simulink model "FlexibleJoint_PD"  (R2019b)
settings: Solver=VariableStepAuto  StartTime=0.0  StopTime=10  RelTol=1e-3
libraries: simulink x3, robotcorelib x1
settings Model: Creator=USER  LastModifiedBy=USER

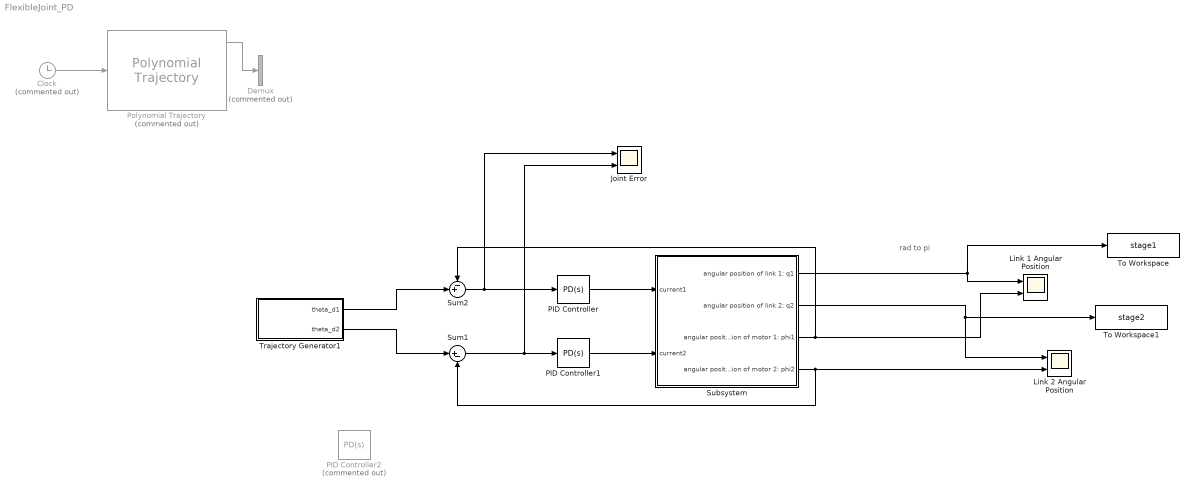
== system FlexibleJoint_PD ==
  note: rad to pi
  Clock : Clock  Commented=on
  Demux : Demux  Commented=on  Outputs=2
  Joint Error : Scope  NumInputPorts=2
  Link 1 Angular Position : Scope  NumInputPorts=2
  Link 2 Angular Position : Scope  NumInputPorts=2
  PID Controller : simulink/Continuous/PID Controller  Controller=PD  Form=Parallel  TimeDomain=Continuous-time  SampleTime=-1  IntegratorMethod=Forward Euler  FilterMethod=Forward Euler  ControllerParametersSource=internal  P=0.6  I=0.00248207984793386  D=0.05  UseFilter=on  N=100  TunerSelectOption=Transfer Function Based (PID Tuner App)  InitialConditionSource=internal  InitialConditionForIntegrator=0  InitialConditionForFilter=0  DifferentiatorICPrevScaledInput=0  ExternalReset=none  TrackingMode=off  Kt=1  LimitOutput=off  UpperSaturationLimit=inf  LowerSaturationLimit=-inf  LinearizeAsGain=on  AntiWindupMode=none  Kb=1  POutMin=[]  POutMax=[]  IOutMin=[]  IOutMax=[]  DOutMin=[]  DOutMax=[]  NOutMin=[]  NOutMax=[]  SumOutMin=[]  SumOutMax=[]  SaturationOutMin=[]  SaturationOutMax=[]  PParamMin=[]  PParamMax=[]  IParamMin=[]  IParamMax=[]  DParamMin=[]  DParamMax=[]  NParamMin=[]  NParamMax=[]  KbParamMin=[]  KbParamMax=[]  KtParamMin=[]  KtParamMax=[]  KbOutMin=[]  KbOutMax=[]  KtOutMin=[]  KtOutMax=[]  IntegratorOutMin=[]  IntegratorOutMax=[]  FilterOutMin=[]  FilterOutMax=[]  SumI1OutMin=[]  SumI1OutMax=[]  SumI2OutMin=[]  SumI2OutMax=[]  SumI3OutMin=[]  SumI3OutMax=[]  SumI4OutMin=[]  SumI4OutMax=[]  SumDOutMin=[]  SumDOutMax=[]  DifferentiatorOutMin=[]  DifferentiatorOutMax=[]  FilterDiffOutCoefMin=[]  FilterDiffOutCoefMax=[]  ReciprocalOutMin=[]  ReciprocalOutMax=[]  SumDenOutMin=[]  SumDenOutMax=[]  SumNumOutMin=[]  SumNumOutMax=[]  DivideOutMin=[]  DivideOutMax=[]  IntegratorContinuousStateAttributes=''  IntegratorStateMustResolveToSignalObject=off  IntegratorRTWStateStorageClass=Auto  FilterContinuousStateAttributes=''  FilterStateMustResolveToSignalObject=off  FilterRTWStateStorageClass=Auto  ParallelPVariant=InternalParameters  IdealPVariant=Disabled  IVariant=Disabled  DVariant=InternalParameters  IntegratorVariant=Disabled  SatVariant=Disabled  AWVariant=Disabled  PCopyVariant=Disabled  TRVariant=Disabled  FdbkBlocksVariant=Forward  IdealPFdbkVariant=Disabled  SatFdbkVariant=Disabled  DerivativeFilterVariant=ContFilter  NVariant=InternalParameters  NCopyVariant=Disabled  FilterICVariant=InternalICsFilter  IntegratorICVariant=Disabled  ExternalResetVariant=Disabled  TRSumVariant=Passthrough  SumFdbkVariant=Disabled  SumVariant=Sum_PD
  PID Controller1 : simulink/Continuous/PID Controller  Controller=PD  Form=Parallel  TimeDomain=Continuous-time  SampleTime=-1  IntegratorMethod=Forward Euler  FilterMethod=Forward Euler  ControllerParametersSource=internal  P=0.65  I=0.00248207984793386  D=0.05  UseFilter=on  N=100  TunerSelectOption=Transfer Function Based (PID Tuner App)  InitialConditionSource=internal  InitialConditionForIntegrator=0  InitialConditionForFilter=0  DifferentiatorICPrevScaledInput=0  ExternalReset=none  TrackingMode=off  Kt=1  LimitOutput=off  UpperSaturationLimit=inf  LowerSaturationLimit=-inf  LinearizeAsGain=on  AntiWindupMode=none  Kb=1  POutMin=[]  POutMax=[]  IOutMin=[]  IOutMax=[]  DOutMin=[]  DOutMax=[]  NOutMin=[]  NOutMax=[]  SumOutMin=[]  SumOutMax=[]  SaturationOutMin=[]  SaturationOutMax=[]  PParamMin=[]  PParamMax=[]  IParamMin=[]  IParamMax=[]  DParamMin=[]  DParamMax=[]  NParamMin=[]  NParamMax=[]  KbParamMin=[]  KbParamMax=[]  KtParamMin=[]  KtParamMax=[]  KbOutMin=[]  KbOutMax=[]  KtOutMin=[]  KtOutMax=[]  IntegratorOutMin=[]  IntegratorOutMax=[]  FilterOutMin=[]  FilterOutMax=[]  SumI1OutMin=[]  SumI1OutMax=[]  SumI2OutMin=[]  SumI2OutMax=[]  SumI3OutMin=[]  SumI3OutMax=[]  SumI4OutMin=[]  SumI4OutMax=[]  SumDOutMin=[]  SumDOutMax=[]  DifferentiatorOutMin=[]  DifferentiatorOutMax=[]  FilterDiffOutCoefMin=[]  FilterDiffOutCoefMax=[]  ReciprocalOutMin=[]  ReciprocalOutMax=[]  SumDenOutMin=[]  SumDenOutMax=[]  SumNumOutMin=[]  SumNumOutMax=[]  DivideOutMin=[]  DivideOutMax=[]  IntegratorContinuousStateAttributes=''  IntegratorStateMustResolveToSignalObject=off  IntegratorRTWStateStorageClass=Auto  FilterContinuousStateAttributes=''  FilterStateMustResolveToSignalObject=off  FilterRTWStateStorageClass=Auto  ParallelPVariant=InternalParameters  IdealPVariant=Disabled  IVariant=Disabled  DVariant=InternalParameters  IntegratorVariant=Disabled  SatVariant=Disabled  AWVariant=Disabled  PCopyVariant=Disabled  TRVariant=Disabled  FdbkBlocksVariant=Forward  IdealPFdbkVariant=Disabled  SatFdbkVariant=Disabled  DerivativeFilterVariant=ContFilter  NVariant=InternalParameters  NCopyVariant=Disabled  FilterICVariant=InternalICsFilter  IntegratorICVariant=Disabled  ExternalResetVariant=Disabled  TRSumVariant=Passthrough  SumFdbkVariant=Disabled  SumVariant=Sum_PD
  PID Controller2 : simulink/Continuous/PID Controller  Commented=on  Controller=PD  Form=Parallel  TimeDomain=Continuous-time  SampleTime=-1  IntegratorMethod=Forward Euler  FilterMethod=Forward Euler  ControllerParametersSource=internal  P=0.8  I=0.00248207984793386  D=0.05  UseFilter=on  N=100  TunerSelectOption=Transfer Function Based (PID Tuner App)  InitialConditionSource=internal  InitialConditionForIntegrator=0  InitialConditionForFilter=0  DifferentiatorICPrevScaledInput=0  ExternalReset=none  TrackingMode=off  Kt=1  LimitOutput=off  UpperSaturationLimit=inf  LowerSaturationLimit=-inf  LinearizeAsGain=on  AntiWindupMode=none  Kb=1  POutMin=[]  POutMax=[]  IOutMin=[]  IOutMax=[]  DOutMin=[]  DOutMax=[]  NOutMin=[]  NOutMax=[]  SumOutMin=[]  SumOutMax=[]  SaturationOutMin=[]  SaturationOutMax=[]  PParamMin=[]  PParamMax=[]  IParamMin=[]  IParamMax=[]  DParamMin=[]  DParamMax=[]  NParamMin=[]  NParamMax=[]  KbParamMin=[]  KbParamMax=[]  KtParamMin=[]  KtParamMax=[]  KbOutMin=[]  KbOutMax=[]  KtOutMin=[]  KtOutMax=[]  IntegratorOutMin=[]  IntegratorOutMax=[]  FilterOutMin=[]  FilterOutMax=[]  SumI1OutMin=[]  SumI1OutMax=[]  SumI2OutMin=[]  SumI2OutMax=[]  SumI3OutMin=[]  SumI3OutMax=[]  SumI4OutMin=[]  SumI4OutMax=[]  SumDOutMin=[]  SumDOutMax=[]  DifferentiatorOutMin=[]  DifferentiatorOutMax=[]  FilterDiffOutCoefMin=[]  FilterDiffOutCoefMax=[]  ReciprocalOutMin=[]  ReciprocalOutMax=[]  SumDenOutMin=[]  SumDenOutMax=[]  SumNumOutMin=[]  SumNumOutMax=[]  DivideOutMin=[]  DivideOutMax=[]  IntegratorContinuousStateAttributes=''  IntegratorStateMustResolveToSignalObject=off  IntegratorRTWStateStorageClass=Auto  FilterContinuousStateAttributes=''  FilterStateMustResolveToSignalObject=off  FilterRTWStateStorageClass=Auto  ParallelPVariant=InternalParameters  IdealPVariant=Disabled  IVariant=Disabled  DVariant=InternalParameters  IntegratorVariant=Disabled  SatVariant=Disabled  AWVariant=Disabled  PCopyVariant=Disabled  TRVariant=Disabled  FdbkBlocksVariant=Forward  IdealPFdbkVariant=Disabled  SatFdbkVariant=Disabled  DerivativeFilterVariant=ContFilter  NVariant=InternalParameters  NCopyVariant=Disabled  FilterICVariant=InternalICsFilter  IntegratorICVariant=Disabled  ExternalResetVariant=Disabled  TRSumVariant=Passthrough  SumFdbkVariant=Disabled  SumVariant=Sum_PD
  Polynomial Trajectory : robotcorelib/Polynomial Trajectory  Commented=on  WaypointSource=Internal  Waypoints=[ 0, pi/4; 0, pi/4]  TimePoints=[ 0, 4]  TimeInterval=[ 1, 4 ]  Method=Cubic Polynomial  ParameterSource=Internal  VelocityBoundaryCondition=zeros( 2, 2 )  AccelerationBoundaryCondition=zeros( 2, 5 )  SimulateUsing=Interpreted execution
      settings: SourceProductName=Robotics System Toolbox  SourceProductBaseCode=RO
  Subsystem : Subsystem
  Sum1 : Sum  Inputs=|+-
  Sum2 : Sum  Inputs=-+|
  To Workspace : ToWorkspace  VariableName=stage1  SaveFormat=Timeseries  SampleTime=-1
  To Workspace1 : ToWorkspace  VariableName=stage2  SaveFormat=Timeseries  SampleTime=-1
  Trajectory Generator1 : MATLAB Function  TreatAsAtomicUnit=on
  wires:
  Subsystem/2(angular position of link 2: q2) -> Link 2 Angular Position/1, To Workspace1/1
  Subsystem/1(angular position of link 1: q1) -> Link 1 Angular Position/1, To Workspace/1
  PID Controller1/1 -> Subsystem/2("current2 ")
  Subsystem/4(angular position of motor 2: phi2) -> Link 2 Angular Position/2, Sum1/2
  Sum2/1 -> Joint Error/1, PID Controller/1
  Subsystem/3(angular position of motor 1: phi1) -> Sum2/1, Link 1 Angular Position/2
  Sum1/1 -> PID Controller1/1, Joint Error/2
  PID Controller/1 -> Subsystem/1(current1)
  Trajectory Generator1/1(theta_d1) -> Sum2/2
  Trajectory Generator1/2(theta_d2) -> Sum1/1
  Polynomial Trajectory/1 -> Demux/1
  Clock/1 -> Polynomial Trajectory/1

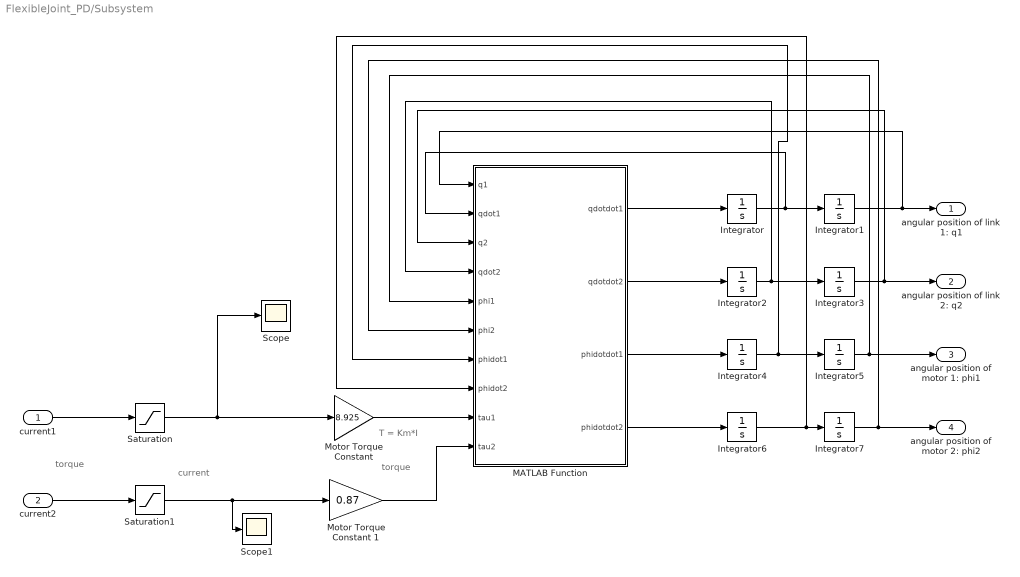
== system FlexibleJoint_PD/Subsystem ==
  note: current
  note: torque
  note: T = Km*I
  note: torque
  current1 : Inport
  "current2 " : Inport  Port=2
  Integrator{,1..7} (8 alike) : Integrator
  MATLAB Function : MATLAB Function  TreatAsAtomicUnit=on
  "Motor Torque Constant " : Gain  Gain=8.925
  Motor Torque Constant 1 : Gain  Gain=0.87
  Saturation : Saturate  UpperLimit=1  LowerLimit=-1
  Saturation1 : Saturate
  Scope : Scope
  Scope1 : Scope
  angular position of link 1: q1 : Outport
  angular position of link 2: q2 : Outport  Port=2
  angular position of motor 1: phi1 : Outport  Port=3
  angular position of motor 2: phi2 : Outport  Port=4
  wires:
  Integrator2/1 -> Integrator3/1, MATLAB Function/4(qdot2)
  Integrator7/1 -> MATLAB Function/6(phi2), angular position of motor 2: phi2/1
  Integrator3/1 -> angular position of link 2: q2/1, MATLAB Function/3(q2)
  Integrator1/1 -> angular position of link 1: q1/1, MATLAB Function/1(q1)
  Integrator/1 -> MATLAB Function/2(qdot1), Integrator1/1
  Saturation1/1 -> Scope1/1, Motor Torque Constant 1/1
  Integrator6/1 -> MATLAB Function/8(phidot2), Integrator7/1
  Integrator4/1 -> Integrator5/1, MATLAB Function/7(phidot1)
  MATLAB Function/2(qdotdot2) -> Integrator2/1
  MATLAB Function/3(phidotdot1) -> Integrator4/1
  Integrator5/1 -> angular position of motor 1: phi1/1, MATLAB Function/5(phi1)
  MATLAB Function/4(phidotdot2) -> Integrator6/1
  "Motor Torque Constant "/1 -> MATLAB Function/9(tau1)
  MATLAB Function/1(qdotdot1) -> Integrator/1
  Motor Torque Constant 1/1 -> MATLAB Function/10(tau2)
  Saturation/1 -> Scope/1, "Motor Torque Constant "/1
  current1/1 -> Saturation/1
  "current2 "/1 -> Saturation1/1

== matlab function FlexibleJoint_PD/Trajectory Generator1 ==
  data: theta_d1 output; theta_d2 output
function [theta_d1,theta_d2]  = fcn
theta_start1 = 0;
theta_start2 = 0;
theta_end1 = pi/4;
theta_end2 = pi/4;
theta_d1 = theta_start1 + (theta_end1-theta_start1);
theta_d2 = theta_start2 + (theta_end2-theta_start2);

== matlab function FlexibleJoint_PD/Subsystem/MATLAB Function ==
  data: q1 input; qdotdot1 output; qdot1 input; q2 input; qdot2 input; phi1 input; phi2 input; phidot1 input; phidot2 input; tau1 input; tau2 input; qdotdot2 output; phidotdot1 output; phidotdot2 output
function [qdotdot1,qdotdot2,phidotdot1,phidotdot2] = fcn(q1,qdot1,q2,qdot2,phi1,phi2,phidot1,phidot2,tau1,tau2)
%y is thetadotdot
tau = [0;0;tau1;tau2];
%Veltman Thesis Values
% m1 = 0.5; 
% m2 = 1;
% L1 = 0.343;
% L2 = 0.267;
% Lc1 = 0.2;
% Lc2 = 0.25;
% I1 = 0.01;
% I2 = 0.01;
% B1 = 0.070364;
% B2 = 0.028211;

%Electrical School values
L1 = 0.343;
L2 = 0.267;
Lc1 = 0.1590;
Lc2 = 0.0550;
m1 = 1.51;
m2 = 0.87326;
I1 = 0.0392;
I2 = 0.0081;
B1 = 0.070364;
B2 = 0.028211;
Bm1 =4.5;
Bm2 = 0.5;
Ks1 = 9;
Ks2 = 4;
Ir1 = 0.0628;
Ir2 = 0.0026;

z = [0 0;
     0 0];
M11 = I2+I1+m2*((L1^2)+(Lc2^2)+2*L1*Lc2*cos(q2))+m1*(Lc1^2);
M12 = I2+m2*(Lc2^2)+L1*Lc2*m2*cos(q2);
M21 = M12;
M22 = I2+m2*(Lc2^2);

M1 = [M11 M12;
     M21 M22];

M2 = [Ir1 0;
      0 Ir2];
  
M = [M1 z;
     z  M2];
 
C11 = -m2*L1*Lc2*sin(q2)*qdot2;
C12 = -m2*L1*Lc2*sin(q2)*qdot2-m2*L1*Lc2*sin(q2)*qdot1;
C21 = m2*L1*Lc2*sin(q2)*qdot1;
C22 = 0;

Ca = [C11 C12;
     C21 C22];

C = [Ca z;
     z  z];
 
K1 = [Ks1 0;
      0  Ks2];
  
K = [K1 -K1;
     -K1 K1];
 
fvl = [B1 0;
      0  B2];
  
fvm = [Bm1 0;
       0  Bm2];
   
fv = [fvl z;
      z  fvm];
  
fvf = fv*[qdot1;qdot2;phidot1;phidot2];
Cf = C*[qdot1;qdot2;phidot1;phidot2];
Kf = K*[q1;q2;phi1;phi2];

y = inv(M)*(tau-Cf-fvf-Kf);
qdotdot1 = y(1);
qdotdot2 = y(2);
phidotdot1 = y(3);
phidotdot2 = y(4);
